simulink model "MagneticXplorer"  (R2024b)
settings: Solver=FixedStepAuto  StartTime=0.0  StopTime=inf  FixedStep=0.001  RelTol=1e-3  EnableMultiTasking=on
libraries: stm32f4xxblockslib x2
settings Model: STM32="{\"AnalogInput\":{\"ID\":\"MagneticXplorer:4\"},\"DigitalPortRead\":{\"ID\":\"MagneticXplorer:28\"}}"  Creator=Lenovo  LastModifiedBy=Lenovo
settings OptimizationCC: DefaultParameterBehavior=Inlined  EnhancedBackFolding=on  PassReuseOutputArgsAs=Individual arguments  ZeroExternalMemoryAtStartup=off  ZeroInternalMemoryAtStartup=off  MaxStackSize=512  OptimizeBlockOrder=speed  DifferentSizesBufferReuse=on  OptimizationCustomize=off  EfficientTunableParamExpr=on
settings DebuggingCC: ParameterTunabilityLossMsg=error
settings HardwareCC: ProdBitPerPointer=32  ProdBitPerSizeT=32  ProdBitPerPtrDiffT=32  ProdLargestAtomicInteger=Long  ProdLargestAtomicFloat=Double  ProdWordSize=32  ProdLongLongMode=on  ProdHWDeviceType=ARM Compatible->ARM Cortex-M
settings SFSimCC: MATLABDynamicMemAlloc=off
settings RTWCC: Description=Embedded Coder  SystemTargetFile=ert.tlc  HardwareBoard=STM32G4xx Based  TemplateMakefile=ert_default_tmf  Toolchain=GNU Tools for ARM Embedded Processors
settings CodeAppCC: ForceParamTrailComments=on  IgnoreCustomStorageClasses=off  OperatorAnnotations=on  SimulinkDataObjDesc=on  SFDataObjDesc=on  InsertBlockDesc=on
settings ERTTargetCC: TargetLangStandard=C99 (ISO)  CodeReplacementLibrary=ARM Cortex-M  ExtModeTransport=3  ExtModeStaticAlloc=on  ExtModeStaticAllocSize=2048  ExtModeMexFile=ext_xcp  ExtModeIntrfLevel=Level2 - Open

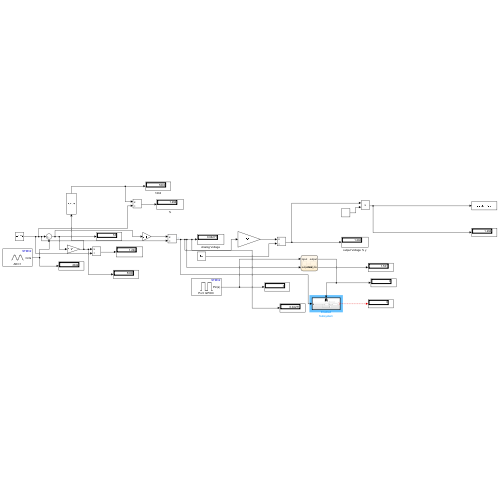
[thumbnail: Simulink's stored preview of the top-level diagram]
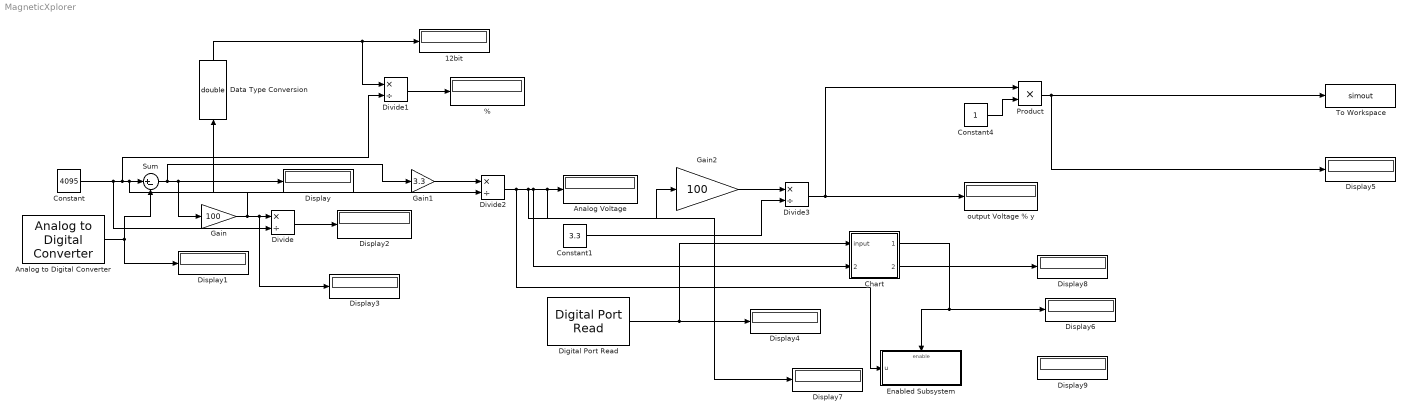
== system MagneticXplorer ==
  % : Display
  12bit : Display
  Analog Voltage : Display
  Analog to Digital Converter : stm32f4xxblockslib/Analog to Digital Converter  ADCModule=ADC1  ConversionGroup=Regular  TriggerMode=Trigger and read  NumberOfConversions=1  EnableBufferConv=off  BufferLength=1  OutputStatus=off  SampleTime=-1  EnableSimPort=off  hoistedMaskSrc=ECSoC/ECSimCodegen/Analog to Digital Converter
  Chart : Stateflow chart  TreatAsAtomicUnit=on
  Constant : Constant  Value=4095
  Constant1 : Constant  Value=3.3
  Constant4 : Constant
  Data Type Conversion : DataTypeConversion  OutDataTypeStr=double  RndMeth=Floor
  Digital Port Read : stm32f4xxblockslib/Digital Port Read  PortName=GPIOC  PinNumber=[13]  ReadOperation=on  IOAsArray=on  SampleTime=-1  EnableSimPort=off  hoistedMaskSrc=ECSoC/ECSimCodegen/Digital Port Read
      settings: LibrarySourceBlock=stm32g4xxblockslib/Digital Port Read
  Display{,1..9} (10 alike) : Display
  Divide{,1..3} (4 alike) : Product  Inputs=*/
  Enabled Subsystem : Subsystem  TreatAsAtomicUnit=on
  Gain : Gain  Gain=100
  Gain1 : Gain  Gain=3.3
  Gain2 : Gain  Gain=100
  Product : Product
  Sum : Sum  Inputs=|+-
  To Workspace : ToWorkspace  VariableName=simout  SampleTime=-1
  output Voltage % y : Display
  wires:
  Constant4/1 -> Product/2
  Divide2/1 -> Enabled Subsystem/1(u), Gain2/1, Chart/2(outputvolt), Display7/1, Analog Voltage/1
  Product/1 -> Display5/1, To Workspace/1
  Gain2/1 -> Divide3/1
  Data Type Conversion/1 -> Divide1/1, 12bit/1
  Divide3/1 -> Product/1, output Voltage % y/1
  Divide/1 -> Display2/1
  Gain1/1 -> Divide2/1
  Divide1/1 -> %/1
  Analog to Digital Converter/1 -> Sum/2, Display1/1
  Constant/1 -> Divide/2, Divide1/2, Divide2/2, Sum/1
  Sum/1 -> Gain1/1, Gain/1, Display/1
  Constant1/1 -> Divide3/2
  Gain/1 -> Data Type Conversion/1, Display3/1, Divide/1
  Digital Port Read/1 -> Chart/1(input), Display4/1
  Chart/1(output) -> Display6/1, Enabled Subsystem/Enable
  Chart/2(time_dis) -> Display8/1
  ? -> Display9/1

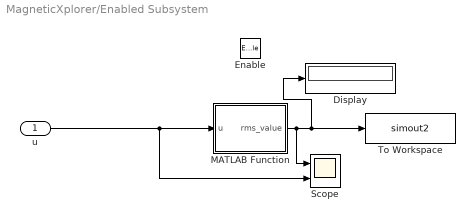
== system MagneticXplorer/Enabled Subsystem ==
  u : Inport
  Enable : EnablePort
  Display : Display
  MATLAB Function : MATLAB Function  TreatAsAtomicUnit=on
  Scope : Scope  NumInputPorts=2
  To Workspace : ToWorkspace  VariableName=simout2  SaveFormat=Timeseries  SampleTime=-1
  wires:
  u/1 -> Scope/2, MATLAB Function/1(u)
  MATLAB Function/1(rms_value) -> Scope/1, Display/1, To Workspace/1

== matlab function MagneticXplorer/Enabled Subsystem/MATLAB Function ==
  data: u input; rms_value output
function rms_value = fcn(u)
    % Get the size of input data u
    n = 1;  % Determine how many elements are in u
    
    % Initialize an array to store the 1000 data points
    persistent data_array;  % Use persistent to store data across function calls
    persistent count;       % To keep track of how many data points have been stored
    
    if isempty(data_array)
        data_array = zeros(1000, 1);  % Preallocate space for 1000 data points
        count = 0;                    % Initialize the count
    end
    
    % Loop through each element of the input data and store it
    for i = 1:n
        if count < 1000
            count = count + 1;
            data_array(count) = u(i);  % Store the data
        end
    end
    
    % Once 1000 data points have been stored, calculate the RMS
    if count == 1000
        % Calculate the RMS value
        rms_value = sqrt(mean(data_array.^2));
        
        % Reset the count and data_array if needed for continuous calculations
        count = 0;
        data_array = zeros(1000, 1);
    else
        rms_value = NaN;  % Output NaN until 1000 points have been collected
    end
    count = 0;  
end

== stateflow chart MagneticXplorer/Chart ==
  state initial
    entry:
    time=0;
    outputvolt;
    output= 0;
  state State
    entry:
    output = 1;
    during:
    time = time + 0.001;
    time_dis = time;
    exit:
    output = 0;
    time = 0;
  (default) -> initial
  initial -> State : [input == 1]
  State -> initial : [time > 1.5]
  data: input input; outputvolt input; output output; time local; time_dis output
